simulink model "Sim_Quadcopter_RL"  (R2021a)
settings: Solver=FixedStepAuto  StartTime=0.0  StopTime=Tf  FixedStep=0.001  RelTol=1e-3
undefined symbols (not defined in the file or in its folder): B, m
libraries: simulink x4, rllib x1, shared6dof x1
settings Model: SimulationMode=accelerator  Creator=ACER  LastModifiedBy=ACER

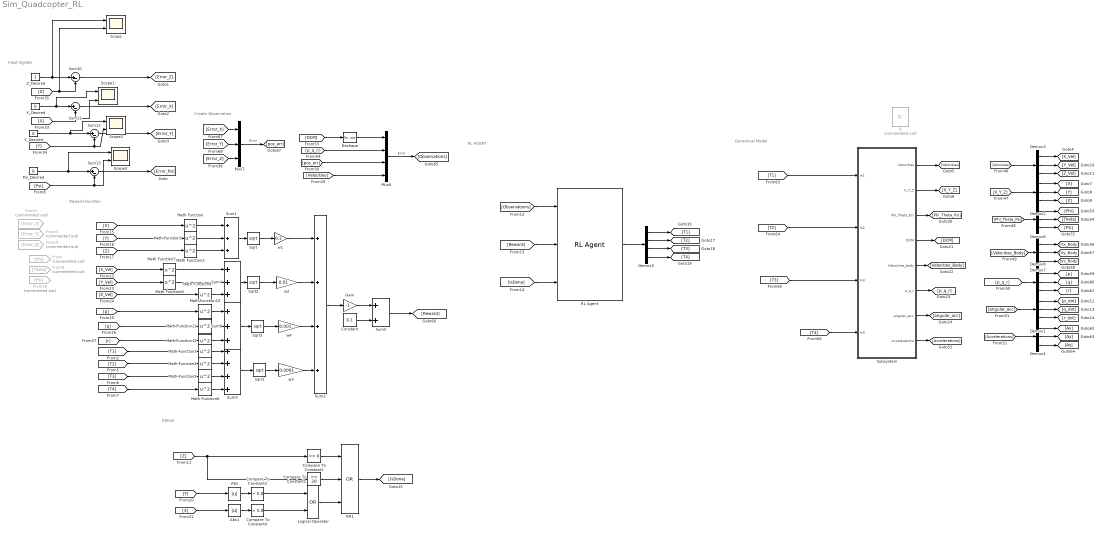
== system Sim_Quadcopter_RL ==
  note: IsDone
  note: Input Signals
  note: Create Observation
  note: Reward Function
  note: Dynamical Model
  note: RL AGENT
  Abs : Abs
  Abs1 : Abs
  Compare To Constant1 : simulink/Logic and Bit Operations/Compare To Constant  relop=<=  const=0  OutDataTypeStr=boolean
  Compare To Constant2 : simulink/Logic and Bit Operations/Compare To Constant  relop=>=  const=20  OutDataTypeStr=boolean
  Compare To Constant3 : simulink/Logic and Bit Operations/Compare To Constant  relop=>  const=5.0  OutDataTypeStr=boolean
  Compare To Constant4 : simulink/Logic and Bit Operations/Compare To Constant  relop=>  const=5.0  OutDataTypeStr=boolean
  Constant : Constant  Value=0.1
  Demux{1..4,6..8} (7 alike) : Demux  Outputs=3
  Demux5 : Demux
  From : From  Commented=on  GotoTag=Phi
  From1 : From  Commented=on  GotoTag=Error_X
  From10 : From  Commented=on  GotoTag=Psi
  From3 : From  Commented=on  GotoTag=Error_Y
  From4 : From  Commented=on  GotoTag=Error_Z
  From9 : From  Commented=on  GotoTag=Theta
  Gain : Gain  Gain=-1
  IC : InitialCondition  Commented=on
  Logical Operator : Logic  Operator=OR  AllPortsSameDT=off
  Math Function{,1..12} (13 alike) : Math  Operator=square  SaturateOnIntegerOverflow=on
  Mux6 : Mux
  Mux7 : Mux  Inputs=3
  OR1 : Logic  Operator=OR  Inputs=3  AllPortsSameDT=off  OutDataTypeStr=boolean
  Psi_Desired : Constant  Value=0
  RL Agent : rllib/RL Agent  Agent=agent  ExternalActionAsInput=off  ProvideCumRwd=off  TreatAsDirectFeedthrough=on
  Reshape : Reshape
  Scope{,1..3} (4 alike) : Scope  NumInputPorts=2
  Sqrt{,1..3} (4 alike) : Sqrt  SaturateOnIntegerOverflow=on
  Subsystem : Subsystem
  Sum1 : Sum  Inputs=+++
  Sum{10..13} (4 alike) : Sum  Inputs=|+-
  Sum2 : Sum  Inputs=++++
  Sum3 : Sum  Inputs=++++
  Sum4 : Sum  Inputs=+++
  Sum5 : Sum
  Sum6 : Sum  Inputs=+++
  X_Desired : Constant  Value=0
  Y_Desired : Constant  Value=0
  Z_Desired : Constant
  w1 : Gain  Gain=0.1
  w2 : Gain  Gain=0.01
  w3 : Gain  Gain=0.0001
  w4 : Gain  Gain=0.001
  wires:
  [T1] -> Subsystem/1(In1)
  [T2] -> Subsystem/2(In2)
  [T3] -> Subsystem/3(In3)
  [T4] -> Subsystem/4(In4)
  Subsystem/2(X_Y_Z) -> [X_Y_Z]
  Subsystem/1(Velocities) -> [Velocities]
  Demux2/1 -> [X]
  Demux2/2 -> [Y]
  Demux2/3 -> [Z]
  X_Desired/1 -> Scope1/1, Sum11/1
  Sum12/1 -> [Error_Y]
  Demux3/1 -> [X_Vel]
  Demux3/2 -> [Y_Vel]
  Demux3/3 -> [Z_Vel]
  Z_Desired/1 -> Scope/1, Sum10/1
  [Observations] -> RL Agent/1
  [Reward] -> RL Agent/2
  [IsDone] -> RL Agent/3
  RL Agent/1 -> Demux5/1
  Psi_Desired/1 -> Scope3/1, Sum13/1
  Demux5/1 -> [T1]
  Demux5/2 -> [T2]
  Demux5/3 -> [T3]
  Demux5/4 -> [T4]
  Subsystem/3(Phi_Theta_Psi) -> [Phi_Theta_Psi]
  [Velocities] -> Demux3/1
  [X_Y_Z] -> Demux2/1
  Subsystem/4(DCM) -> [DCM]
  Subsystem/5(Velocities_body) -> [Velocities_Body]
  Subsystem/6(p_q_r) -> [p_q_r]
  Subsystem/7(angular_acc) -> [angular_acc]
  Subsystem/8(Accelerations) -> [Accelerations]
  [Phi_Theta_Psi] -> Demux6/1
  Demux6/1 -> [Phi]
  Demux6/2 -> [Theta]
  Demux6/3 -> [Psi]
  [Velocities_Body] -> Demux7/1
  Demux7/1 -> [Vx_Body]
  Demux7/2 -> [Vy_Body]
  Demux7/3 -> [Vz_Body]
  [p_q_r] -> Demux8/1
  Demux8/1 -> [p]
  Demux8/2 -> [q]
  Demux8/3 -> [r]
  [angular_acc] -> Demux1/1
  Demux1/1 -> [p_dot]
  Demux1/2 -> [q_dot]
  Demux1/3 -> [r_dot]
  [Accelerations] -> Demux4/1
  Demux4/1 -> [Ax]
  Demux4/3 -> [Az]
  Demux4/2 -> [Ay]
  [Velocities] -> Mux6/4
  [p_q_r] -> Mux6/2
  [DCM] -> Reshape/1
  Mux6/1 -> [Observations]  "Error"
  [Z] -> Scope/2, Sum10/2
  Sum10/1 -> [Error_Z]
  [X] -> Scope1/2, Sum11/2
  Sum11/1 -> [Error_X]
  Y_Desired/1 -> Scope2/1, Sum12/1
  [Y] -> Scope2/2, Sum12/2
  [Error_Y] -> Mux7/2
  [Error_X] -> Mux7/1
  [Error_Z] -> Mux7/3
  Mux7/1 -> [pos_err]  "Error"
  [Psi] -> Sum13/2, Scope3/2
  Sum13/1 -> [Error_Psi]
  Sqrt2/1 -> w2/1
  Sum2/1 -> Gain/1
  Gain/1 -> Sum5/1
  [X] -> Math Function/1
  [Y] -> Math Function1/1
  [Z] -> Math Function2/1
  Sum1/1 -> Sqrt/1
  w1/1 -> Sum2/1
  w2/1 -> Sum2/2
  [T1] -> Math Function3/1
  [T2] -> Math Function4/1
  [T3] -> Math Function5/1
  [T4] -> Math Function6/1
  Sum3/1 -> Sqrt1/1
  w3/1 -> Sum2/4
  Math Function/1 -> Sum1/1
  Math Function1/1 -> Sum1/2
  Math Function2/1 -> Sum1/3
  Sqrt/1 -> w1/1
  Math Function3/1 -> Sum3/1
  Math Function4/1 -> Sum3/2
  Math Function5/1 -> Sum3/3
  Math Function6/1 -> Sum3/4
  Sqrt1/1 -> w3/1
  [X_Vel] -> Math Function7/1
  [Y_Vel] -> Math Function8/1
  [Z_Vel] -> Math Function9/1
  Math Function7/1 -> Sum4/1
  Math Function8/1 -> Sum4/2
  Math Function9/1 -> Sum4/3
  Sum4/1 -> Sqrt2/1
  [Z] -> Compare To Constant2/1, Compare To Constant1/1
  Compare To Constant1/1 -> OR1/1
  Compare To Constant2/1 -> OR1/2
  [pos_err] -> Mux6/3
  Reshape/1 -> Mux6/1
  Compare To Constant3/1 -> Logical Operator/1
  Compare To Constant4/1 -> Logical Operator/2
  Abs1/1 -> Compare To Constant4/1
  Abs/1 -> Compare To Constant3/1
  [Y] -> Abs/1
  [X] -> Abs1/1
  Logical Operator/1 -> OR1/3
  Sum5/1 -> [Reward]
  Constant/1 -> Sum5/2
  [p] -> Math Function10/1
  [q] -> Math Function11/1
  [r] -> Math Function12/1
  Math Function12/1 -> Sum6/3
  Math Function11/1 -> Sum6/2
  Math Function10/1 -> Sum6/1
  Sum6/1 -> Sqrt3/1
  Sqrt3/1 -> w4/1
  w4/1 -> Sum2/3
  OR1/1 -> [IsDone]

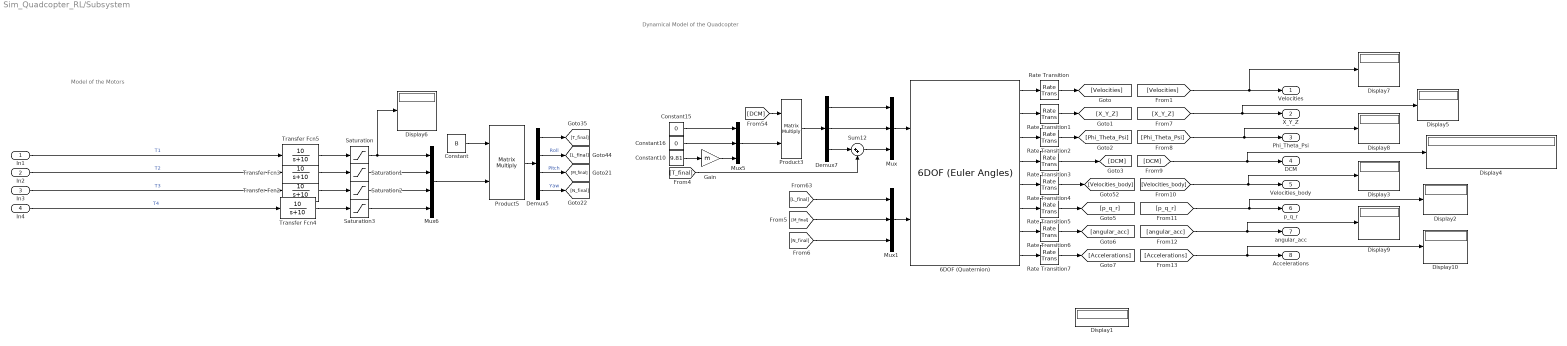
== system Sim_Quadcopter_RL/Subsystem ==
  note: Model of the Motors
  note: Dynamical Model of the Quadcopter
  In1 : Inport
  In2 : Inport  Port=2
  In3 : Inport  Port=3
  In4 : Inport  Port=4
  6DOF (Quaternion) : shared6dof/6DOF (Euler Angles)  units=Metric (MKS)  mtype=Fixed  rep=Quaternion  xme_0=[0 0 0]  Vm_0=[0 0 0]  eul_0=[0 0 0]  pm_0=[0 0 0]  mass_0=0.068  mass_e=0.5  mass_f=2.0  inertia=[0.0686*10^-3 0 0; 0 0.092*10^-3 0;0 0 0.1366*10^-3]  inertia_e=eye(3)  inertia_f=2*eye(3)  k_quat=1.0  vre_flag=on  abi_flag=off  aMode=0  xme_statename=''  Vm_statename=''  eul_statename=''  quat_statename=''  pm_statename=''  mass_statename=''
      settings: SourceProductBaseCode=AE
  Constant : Constant  Value=B
  Constant10 : Constant  Value=9.81
  Constant15 : Constant  Value=0
  Constant16 : Constant  Value=0
  Demux5 : Demux
  Demux7 : Demux  Outputs=3
  Display{1..10} (10 alike) : Display
  Gain : Gain  Gain=m
  Mux : Mux  Inputs=3
  Mux1 : Mux  Inputs=3
  Mux5 : Mux  Inputs=3
  Mux6 : Mux
  Product3 : Product  Multiplication=Matrix(*)
  Product5 : Product  Multiplication=Matrix(*)
  Rate Transition{,1..7} (8 alike) : RateTransition  OutPortSampleTime=0.02
  Saturation{,1..3} (4 alike) : Saturate  UpperLimit=500  LowerLimit=0
  Sum12 : Sum  Inputs=|++
  Transfer Fcn{2..5} (4 alike) : TransferFcn  Numerator=[10]  Denominator=[1 10]
  Velocities : Outport
  X_Y_Z : Outport  Port=2
  Phi_Theta_Psi : Outport  Port=3
  DCM : Outport  Port=4
  Velocities_body : Outport  Port=5
  p_q_r : Outport  Port=6
  angular_acc : Outport  Port=7
  Accelerations : Outport  Port=8
  wires:
  6DOF (Quaternion)/5 -> Rate Transition4/1
  Rate Transition2/1 -> [Phi_Theta_Psi]
  Demux7/3 -> Sum12/1
  Constant/1 -> Product5/1
  Demux7/1 -> Mux/1
  Mux5/1 -> Product3/2
  [Phi_Theta_Psi] -> Display8/1, Phi_Theta_Psi/1
  6DOF (Quaternion)/6 -> Rate Transition5/1
  6DOF (Quaternion)/1 -> Rate Transition/1
  6DOF (Quaternion)/2 -> Rate Transition1/1
  Rate Transition4/1 -> [Velocities_body]
  Rate Transition6/1 -> [angular_acc]
  Product5/1 -> Demux5/1
  6DOF (Quaternion)/4 -> Rate Transition3/1
  Constant16/1 -> Mux5/2
  Demux5/1 -> [T_final]
  Transfer Fcn4/1 -> Saturation3/1
  Demux7/2 -> Mux/2
  Mux/1 -> 6DOF (Quaternion)/1
  Transfer Fcn2/1 -> Saturation2/1
  6DOF (Quaternion)/7 -> Rate Transition6/1
  Saturation3/1 -> Mux6/4
  [DCM] -> Display4/1, DCM/1
  [L_final] -> Mux1/1
  Rate Transition3/1 -> [DCM]
  Rate Transition/1 -> [Velocities]
  Saturation/1 -> Display6/1, Mux6/1
  6DOF (Quaternion)/8 -> Rate Transition7/1
  [N_final] -> Mux1/3
  [Accelerations] -> Display10/1, Accelerations/1
  Rate Transition1/1 -> [X_Y_Z]
  [M_final] -> Mux1/2
  Gain/1 -> Mux5/3
  Product3/1 -> Demux7/1
  Mux6/1 -> Product5/2
  [T_final] -> Sum12/2
  Saturation2/1 -> Mux6/3
  Demux5/4 -> [N_final]  "Yaw"
  Transfer Fcn3/1 -> Saturation1/1
  [X_Y_Z] -> Display5/1, X_Y_Z/1
  6DOF (Quaternion)/3 -> Rate Transition2/1
  Rate Transition5/1 -> [p_q_r]
  Saturation1/1 -> Mux6/2
  Constant10/1 -> Gain/1
  Demux5/3 -> [M_final]  "Pitch"
  Sum12/1 -> Mux/3
  [DCM] -> Product3/1
  Constant15/1 -> Mux5/1
  Transfer Fcn5/1 -> Saturation/1
  Mux1/1 -> 6DOF (Quaternion)/2
  Demux5/2 -> [L_final]  "Roll"
  [Velocities_body] -> Display3/1, Velocities_body/1
  [p_q_r] -> Display2/1, p_q_r/1
  In3/1 -> Transfer Fcn2/1  "T3"
  [angular_acc] -> Display9/1, angular_acc/1
  In2/1 -> Transfer Fcn3/1  "T2"
  In1/1 -> Transfer Fcn5/1  "T1"
  In4/1 -> Transfer Fcn4/1  "T4"
  Rate Transition7/1 -> [Accelerations]
  [Velocities] -> Display7/1, Velocities/1
